simulink model "Dynamic_PMSM"  (R2020a)
settings: Solver=ode4  StartTime=0.0  StopTime=4  FixedStep=1e-4  RelTol=1e-3
PreLoadFcn:
  | % motor parameters
  | rs = 0.2;               %Stator resistance
  | Lq = 300e-6;            %d and q axis inductances
  | Ld = 300e-6;
  | Lambda_m_r = 0.01;      %rotor flux linkages (back-emf constant)
  | P=2;                    % numer of poles
  | % current controller gains
  | BW = 2*pi*(100*0.1592*0.7071); %controller bandwidth in radps
  | Kp = BW*Lq;
  | Ki = BW*rs;
settings Model: Creator=samee
settings DebuggingCC: UnconnectedInputMsg=none  UnconnectedOutputMsg=none  UnconnectedLineMsg=none

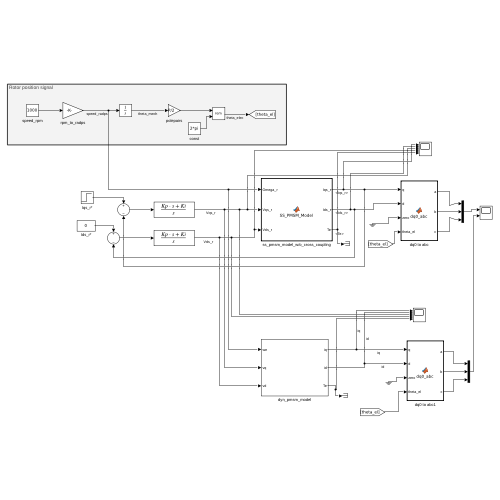
[thumbnail: Simulink's stored preview of the top-level diagram]
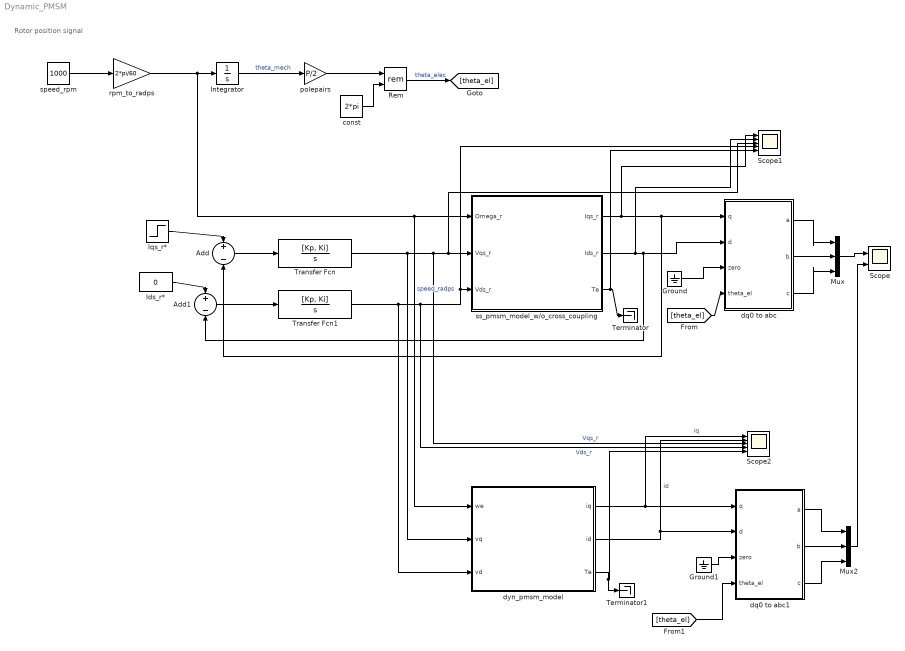
== system Dynamic_PMSM ==
  note: Rotor position signal
  Add : Sum  Inputs=+-
  Add1 : Sum  Inputs=+-
  Ground : Ground
  Ground1 : Ground
  Ids_r* : Constant  Value=0
  Integrator : Integrator
  Iqs_r* : Step  After=3  SampleTime=0
  Mux : Mux  Inputs=3
  Mux2 : Mux  Inputs=3
  Rem : Math  Operator=rem  SaturateOnIntegerOverflow=on
  Scope : Scope  NumInputPorts=2
  Scope1 : Scope  NumInputPorts=5
  Scope2 : Scope  NumInputPorts=5
  Terminator : Terminator
  Terminator1 : Terminator
  Transfer Fcn : TransferFcn  Numerator=[Kp, Ki]  Denominator=[1 0]
  Transfer Fcn1 : TransferFcn  Numerator=[Kp, Ki]  Denominator=[1 0]
  const : Constant  Value=2*pi
  dq0 to abc : MATLAB Function  TreatAsAtomicUnit=on
  dq0 to abc1 : MATLAB Function  TreatAsAtomicUnit=on
  dyn_pmsm_model : Subsystem
  polepairs : Gain  Gain=P/2
  rpm_to_radps : Gain  Gain=2*pi/60
  speed_rpm : Constant  Value=1000
  ss_pmsm_model_w/o_cross_coupling : MATLAB Function  TreatAsAtomicUnit=on
  wires:
  Integrator/1 -> polepairs/1  "theta_mech"
  const/1 -> Rem/2
  polepairs/1 -> Rem/1
  speed_rpm/1 -> rpm_to_radps/1
  rpm_to_radps/1 -> Integrator/1, dyn_pmsm_model/1(we), ss_pmsm_model_w/o_cross_coupling/1(Omega_r)  "speed_radps"
  Rem/1 -> [theta_el]  "theta_elec"
  Transfer Fcn/1 -> dyn_pmsm_model/2(vq), Scope2/3, Scope1/3, ss_pmsm_model_w/o_cross_coupling/2(Vqs_r)  "Vqs_r"
  Transfer Fcn1/1 -> dyn_pmsm_model/3(vd), Scope2/4, Scope1/4, ss_pmsm_model_w/o_cross_coupling/3(Vds_r)  "Vds_r"
  ss_pmsm_model_w/o_cross_coupling/1(Iqs_r) -> Scope1/1, dq0 to abc/1(q), Add/2
  ss_pmsm_model_w/o_cross_coupling/2(Ids_r) -> Scope1/2, dq0 to abc/2(d), Add1/2
  ss_pmsm_model_w/o_cross_coupling/3(Te) -> Scope1/5, Terminator/1
  Ground/1 -> dq0 to abc/3(zero)
  [theta_el] -> dq0 to abc/4(theta_el)
  Iqs_r*/1 -> Add/1
  Add/1 -> Transfer Fcn/1
  Ids_r*/1 -> Add1/1
  Add1/1 -> Transfer Fcn1/1
  dq0 to abc/2(b) -> Mux/2
  dq0 to abc/1(a) -> Mux/1
  dq0 to abc/3(c) -> Mux/3
  Mux/1 -> Scope/1
  dyn_pmsm_model/1(iq) -> Scope2/1, dq0 to abc1/1(q)  "iq"
  dyn_pmsm_model/2(id) -> Scope2/2, dq0 to abc1/2(d)  "id"
  Ground1/1 -> dq0 to abc1/3(zero)
  [theta_el] -> dq0 to abc1/4(theta_el)
  dyn_pmsm_model/3(Te) -> Terminator1/1, Scope2/5
  Mux2/1 -> Scope/2
  dq0 to abc1/3(c) -> Mux2/3
  dq0 to abc1/1(a) -> Mux2/1
  dq0 to abc1/2(b) -> Mux2/2

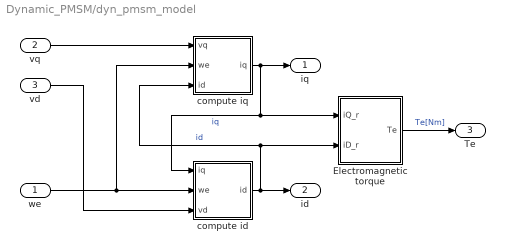
== system Dynamic_PMSM/dyn_pmsm_model ==
  we : Inport
  vq : Inport  Port=2
  vd : Inport  Port=3
  Electromagnetic torque : MATLAB Function  TreatAsAtomicUnit=on
  compute id : Subsystem
  compute iq : Subsystem
  iq : Outport  InitialOutput=0  VectorParamsAs1DForOutWhenUnconnected=off
  id : Outport  Port=2  InitialOutput=0  VectorParamsAs1DForOutWhenUnconnected=off
  Te : Outport  Port=3  InitialOutput=0  VectorParamsAs1DForOutWhenUnconnected=off
  wires:
  compute iq/1(iq) -> compute id/1(iq), Electromagnetic torque/1(iQ_r), iq/1  "iq"
  vq/1 -> compute iq/1(vq)
  vd/1 -> compute id/3(vd)
  we/1 -> compute id/2(we), compute iq/2(we)
  compute id/1(id) -> id/1, compute iq/3(id), Electromagnetic torque/2(iD_r)  "id"
  Electromagnetic torque/1(Te) -> Te/1  "Te[Nm]"

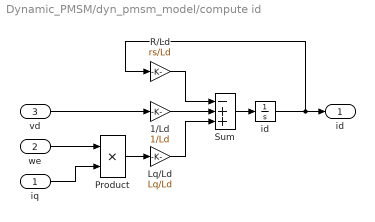
== system Dynamic_PMSM/dyn_pmsm_model/compute id ==
  iq : Inport
  we : Inport  Port=2
  vd : Inport  Port=3
  1/Ld : Gain  Gain=1/Ld  SaturateOnIntegerOverflow=on  OutDataTypeStr=Inherit: Same as input  ParamDataTypeStr=Inherit: Same as input
  Lq/Ld : Gain  Gain=Lq/Ld  SaturateOnIntegerOverflow=on  OutDataTypeStr=Inherit: Same as input  ParamDataTypeStr=Inherit: Same as input
  Product : Product  InputSameDT=on  SaturateOnIntegerOverflow=on  OutDataTypeStr=Inherit: Same as first input
  R/Ld : Gain  Gain=rs/Ld  SaturateOnIntegerOverflow=on  OutDataTypeStr=Inherit: Same as input  ParamDataTypeStr=Inherit: Same as input
  Sum : Sum  Inputs=-++  InputSameDT=on  SaturateOnIntegerOverflow=on  OutDataTypeStr=Inherit: Same as first input
  "id " : Integrator
  id : Outport  InitialOutput=0  VectorParamsAs1DForOutWhenUnconnected=off
  wires:
  1/Ld/1 -> Sum/2
  R/Ld/1 -> Sum/1
  Lq/Ld/1 -> Sum/3
  Sum/1 -> "id "/1
  Product/1 -> Lq/Ld/1
  "id "/1 -> R/Ld/1, id/1
  vd/1 -> 1/Ld/1
  we/1 -> Product/1
  iq/1 -> Product/2

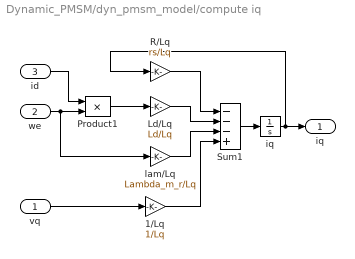
== system Dynamic_PMSM/dyn_pmsm_model/compute iq ==
  vq : Inport
  we : Inport  Port=2
  id : Inport  Port=3
  1/Lq : Gain  Gain=1/Lq  SaturateOnIntegerOverflow=on  OutDataTypeStr=Inherit: Same as input  ParamDataTypeStr=Inherit: Same as input
  Ld/Lq : Gain  Gain=Ld/Lq  SaturateOnIntegerOverflow=on  OutDataTypeStr=Inherit: Same as input  ParamDataTypeStr=Inherit: Same as input
  Product1 : Product  InputSameDT=on  SaturateOnIntegerOverflow=on  OutDataTypeStr=Inherit: Same as first input
  R/Lq : Gain  Gain=rs/Lq  SaturateOnIntegerOverflow=on  OutDataTypeStr=Inherit: Same as input  ParamDataTypeStr=Inherit: Same as input
  Sum1 : Sum  Inputs=---+  InputSameDT=on  SaturateOnIntegerOverflow=on  OutDataTypeStr=Inherit: Same as first input
  "iq " : Integrator
  lam/Lq : Gain  Gain=Lambda_m_r/Lq  SaturateOnIntegerOverflow=on  OutDataTypeStr=Inherit: Same as input  ParamDataTypeStr=Inherit: Same as input
  iq : Outport  InitialOutput=0  VectorParamsAs1DForOutWhenUnconnected=off
  wires:
  R/Lq/1 -> Sum1/1
  Ld/Lq/1 -> Sum1/2
  lam/Lq/1 -> Sum1/3
  Sum1/1 -> "iq "/1
  Product1/1 -> Ld/Lq/1
  1/Lq/1 -> Sum1/4
  id/1 -> Product1/1
  vq/1 -> 1/Lq/1
  we/1 -> Product1/2, lam/Lq/1
  "iq "/1 -> R/Lq/1, iq/1

== matlab function Dynamic_PMSM/dq0 to abc ==
  data: q input; d input; a output; zero input; theta_el input; b output; c output
function [a, b, c] = dq0_abc(q, d, zero, theta_el)

a = cos(theta_el)*q + sin(theta_el)*d + zero*1;
b = cos(theta_el-(2*pi/3))*q + sin(theta_el-(2*pi/3))*d + zero*1;
c = cos(theta_el+(2*pi/3))*q + sin(theta_el+(2*pi/3))*d + zero*1;

== matlab function Dynamic_PMSM/ss_pmsm_model_w//o_cross_coupling ==
  data: Omega_r input; Vqs_r input; Iqs_r output; Vds_r input; Ids_r output; Te output
function [Iqs_r, Ids_r, Te] = SS_PMSM_Model(Omega_r, Vqs_r, Vds_r)
%#codegen

rs = 0.2;               %Stator resistance
Lq = 300e-6;            %d and q axis inductances
Ld = 300e-6;
Lambda_m_r = 0.01;      %rotor flux linkages (back-emf constant)
P=2;                    % numer of poles   


K1 = ((rs^2) + (Omega_r^2)*Ld*Lq);

% Motor currents in rotor reference frame
Iqs_r = (rs/K1) * (Vqs_r - Omega_r*Lambda_m_r - (Omega_r*Ld/rs)*Vds_r);
Ids_r = (1/K1) * (rs*Vds_r + Omega_r*Lq*Vqs_r - (Omega_r^2)*Lq*Lambda_m_r);

% Electromagnetic torque generated
Te = (3/2)*(P/2)*((Lambda_m_r*Iqs_r) + ((Ld - Lq)*Iqs_r*Ids_r));

== matlab function Dynamic_PMSM/dyn_pmsm_model/Electromagnetic torque ==
  data: iQ_r input; Te output; iD_r input
function Te  = Tem(iQ_r, iD_r)
%#codegen

rs = 0.2;               %Stator resistance
Lq = 300e-6;            %d and q axis inductances
Ld = 300e-6;
Lambda_m_r = 0.01;      %rotor flux linkages (back-emf constant)
P=2;                    % numer of poles   


% Electromagnetic torque generated
Te = (3/2)*(P/2)*((Lambda_m_r*iQ_r) + ((Ld - Lq)*iQ_r*iD_r));

== matlab function Dynamic_PMSM/dq0 to abc1 ==
  data: q input; d input; a output; zero input; theta_el input; b output; c output
function [a, b, c] = dq0_abc(q, d, zero, theta_el)

a = cos(theta_el)*q + sin(theta_el)*d + zero*1;
b = cos(theta_el-(2*pi/3))*q + sin(theta_el-(2*pi/3))*d + zero*1;
c = cos(theta_el+(2*pi/3))*q + sin(theta_el+(2*pi/3))*d + zero*1;
